simulink model "bouncing_ball_4"  (R2024a)
settings: Solver=ode45  StartTime=0.0  StopTime=10  RelTol=1e-3  EnableMultiTasking=on
libraries: vrlib x2
settings Model: Creator=smahapat  LastModifiedBy=Miko
settings SolverCC: AlgebraicLoopSolver=TrustRegion
settings DataIOCC: LimitDataPoints=on  SaveFormat=Array  SignalLoggingSaveFormat=ModelDataLogs  ReturnWorkspaceOutputs=off
settings OptimizationCC: ExpressionDepthLimit=2147483647  LifeSpan=inf
settings DebuggingCC: UnderspecifiedInitializationDetection=Classic  MergeDetectMultiDrivingBlocksExec=none  SolverPrmCheckMsg=warning  FcnCallInpInsideContextMsg=warning  UnconnectedInputMsg=warning  UnconnectedOutputMsg=warning  UnconnectedLineMsg=warning  StateNameClashWarn=warning  SFUnexpectedBacktrackingDiag=warning  SFNoUnconditionalDefaultTransitionDiag=warning  SFExecutionAtInitializationDiag=none  ArithmeticOperatorsInVariantConditions=warning
settings HardwareCC: ProdBitPerPointer=32  ProdBitPerSizeT=32  ProdBitPerPtrDiffT=32  ProdLargestAtomicFloat=None  ProdIntDivRoundTo=Undefined  ProdEndianess=Unspecified  ProdWordSize=32  ProdHWDeviceType=32-bit Generic
settings ModelReferenceCC: PropagateSignalLabelsOutOfModel=off
settings SFSimCC: SimUseLocalCustomCode=off  SimParseCustomCode=off  CustomCodeUndefinedFunction=UseInterfaceOnly
settings RTWCC: RTWUseLocalCustomCode=off  GPUComputeCapability=3.5
settings CodeAppCC: StateflowObjectComments=on
settings GRTTargetCC: TargetLangStandard=C89/C90 (ANSI)  CombineOutputUpdateFcns=off  GRTInterface=on
settings ConfigComp: CovMetricSettings=dw  CovSaveCumulativeToWorkspaceVar=on  CovSaveSingleToWorkspaceVar=on  CovExternalEMLEnable=off

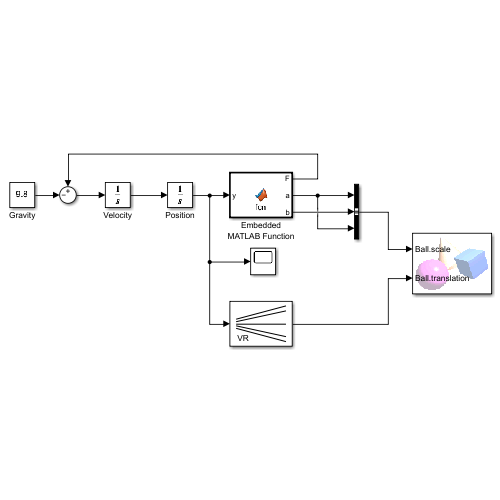
[thumbnail: Simulink's stored preview of the top-level diagram]
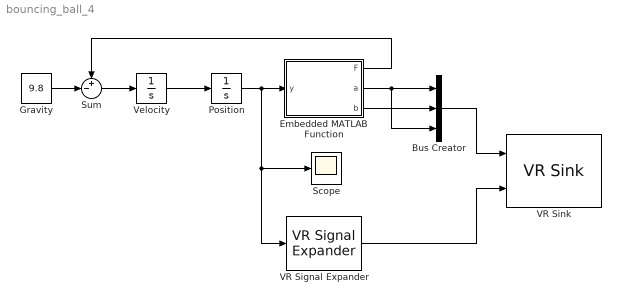
== system bouncing_ball_4 ==
  Bus Creator : BusCreator  Inputs=3
  Embedded MATLAB Function : MATLAB Function  TreatAsAtomicUnit=on
  Gravity : Constant  Value=9.8
  Position : Integrator  InitialCondition=20
  Scope : Scope
  Sum : Sum  Inputs=+-|
  VR Signal Expander : vrlib/VR Signal Expander  outwidth=3  outidx=[2]
  VR Sink : vrlib/VR Sink  InstantiateOnLoad=on  SampleTime=0.01  ViewEnable=on  RemoteChange=off  RemoteView=on  FieldsWritten=Ball.scale.3.1.double#Ball.translation.3.1.double  WorldFileName=bouncing_ball.wrl  AutoView=off  VideoDimensions=[]  AllowVariableSize=off
  Velocity : Integrator
  wires:
  Velocity/1 -> Position/1
  Position/1 -> Embedded MATLAB Function/1(y), VR Signal Expander/1, Scope/1
  Sum/1 -> Velocity/1
  VR Signal Expander/1 -> VR Sink/2
  Bus Creator/1 -> VR Sink/1
  Embedded MATLAB Function/3(b) -> Bus Creator/2
  Embedded MATLAB Function/2(a) -> Bus Creator/1, Bus Creator/3
  Embedded MATLAB Function/1(F) -> Sum/1
  Gravity/1 -> Sum/2

== matlab function bouncing_ball_4/Embedded MATLAB Function ==
  data: F output; a output; b output; y input
function [F,a, b] = fcn(y)
%#eml

if y<1e-4
    y=1e-4;
end

if y<1.5
    f=500*(1.5-y);
    a=sqrt(1.5^3/y);
    b=y;
else
    f=0;
    a=1.5;
    b=1.5;
end
